simulink model "KranModel"  (R2022b)
settings: Solver=ode3  StartTime=0.0  StopTime=10.0  FixedStep=0.001  RelTol=1e-3
values from neighbouring files (symbols this model uses):
  g = 9.81    [KranMfile.m]    (also in V3_Parameter.m)
  i_g = 62    [V3_Parameter.m]
  J = J_m*i_g^2+J_s+m*r_s^2    (= 0.23442)    [V3_Parameter.m]
  k_m = 0.110219939    [V3_Parameter.m]
  KL_REIB = [-2.3005883	-1.712063276	-1.123224093	-0.546846561    -0.001          0.0 0.001 	    0.305048647	0.879017624	1.476234388	2.067272686 ... (first row only)    [V3_Parameter.m]
  L_a = 4.873e-3    (= 0.004873)    [V3_Parameter.m]
  m = 2    [KranMfile.m]    (also in V3_Parameter.m)
  R_a = 2.35    [V3_Parameter.m]
  r_s = 0.1    [V3_Parameter.m]
settings Model: Creator=janbe  LastModifiedBy=JSCHB

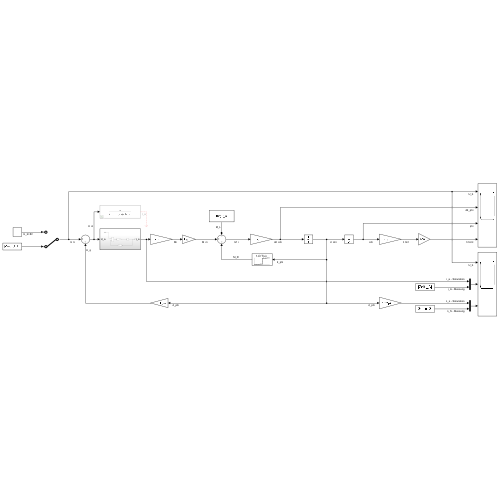
[thumbnail: Simulink's stored preview of the top-level diagram]
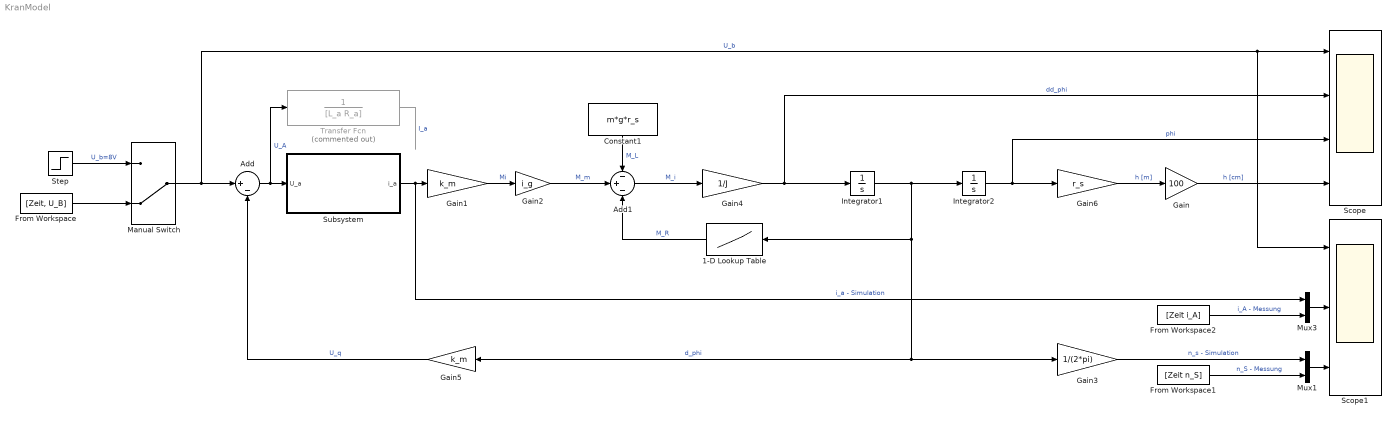
== system KranModel ==
  1-D Lookup Table : Lookup_n-D  NumberOfTableDimensions=1  BreakpointsForDimension1=KL_REIB(1,:)  Table=KL_REIB(2,:)  InternalRulePriority=Speed  RndMeth=Simplest
  Add : Sum  Inputs=|+-
  Add1 : Sum  Inputs=-+-
  Constant1 : Constant  Value=m*g*r_s
  From Workspace : FromWorkspace  VariableName=[Zeit, U_B]
  From Workspace1 : FromWorkspace  VariableName=[Zeit n_S]
  From Workspace2 : FromWorkspace  VariableName=[Zeit i_A]
  Gain : Gain  Gain=100
  Gain1 : Gain  Gain=k_m
  Gain2 : Gain  Gain=i_g
  Gain3 : Gain  Gain=1/(2*pi)
  Gain4 : Gain  Gain=1/J
  Gain5 : Gain  Gain=k_m
  Gain6 : Gain  Gain=r_s
  Integrator1 : Integrator
  Integrator2 : Integrator
  Manual Switch : ManualSwitch  CurrentSetting=0
  Mux1 : Mux  Inputs=2
  Mux3 : Mux  Inputs=2
  Scope : Scope  NumInputPorts=4
  Scope1 : Scope  NumInputPorts=3
  Step : Step  After=8  SampleTime=0
  Subsystem : Subsystem
  Transfer Fcn : TransferFcn  Commented=on  Denominator=[L_a R_a]
  wires:
  Gain1/1 -> Gain2/1  "Mi"
  1-D Lookup Table/1 -> Add1/3  "M_R"
  Constant1/1 -> Add1/1  "M_L"
  Add1/1 -> Gain4/1  "M_i"
  Gain4/1 -> Scope/2, Integrator1/1  "dd_phi"
  Integrator1/1 -> 1-D Lookup Table/1, Gain5/1, Gain3/1, Integrator2/1  "d_phi"
  Integrator2/1 -> Gain6/1, Scope/3  "phi"
  Gain6/1 -> Gain/1  "h [m]"
  Subsystem/1(i_a) -> Mux3/1, Gain1/1  "i_a - Simulation"
  Add/1 -> Transfer Fcn/1, Subsystem/1(U_a)  "U_A"
  Gain5/1 -> Add/2  "U_q"
  Step/1 -> Manual Switch/1  "U_b=8V"
  Transfer Fcn/1 -> ?  "I_a"
  Gain/1 -> Scope/4  "h [cm]"
  Gain2/1 -> Add1/2  "M_m"
  Manual Switch/1 -> Scope/1, Scope1/1, Add/1  "U_b"
  From Workspace/1 -> Manual Switch/2
  Gain3/1 -> Mux1/1  "n_s - Simulation"
  From Workspace1/1 -> Mux1/2  "n_S - Messung"
  Mux1/1 -> Scope1/3
  Mux3/1 -> Scope1/2
  From Workspace2/1 -> Mux3/2  "i_A - Messung"

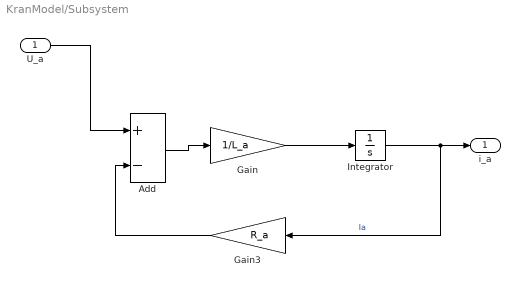
== system KranModel/Subsystem ==
  U_a : Inport
  Add : Sum  Inputs=+-
  Gain : Gain  Gain=1/L_a
  Gain3 : Gain  Gain=R_a
  Integrator : Integrator
  i_a : Outport
  wires:
  U_a/1 -> Add/1
  Gain/1 -> Integrator/1
  Integrator/1 -> i_a/1, Gain3/1  "Ia"
  Add/1 -> Gain/1
  Gain3/1 -> Add/2
